simulink model "Serialising"  (R2024b)
settings: Solver=VariableStepAuto  StartTime=0.0  StopTime=10.0  RelTol=1e-3
model workspace (MAT data in the model file):
  R = 1000
libraries: hdlsllib x2
settings Model: Creator=daniel  LastModifiedBy=daniel

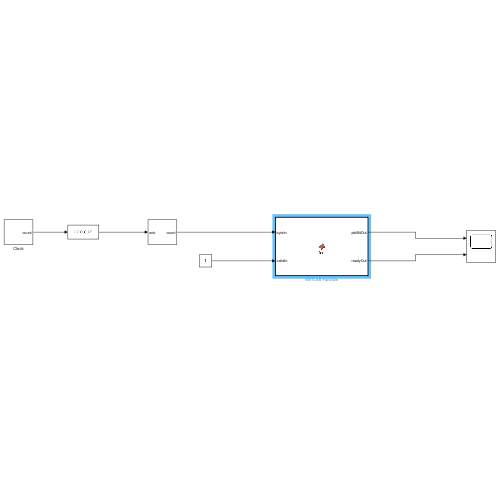
[thumbnail: Simulink's stored preview of the top-level diagram]
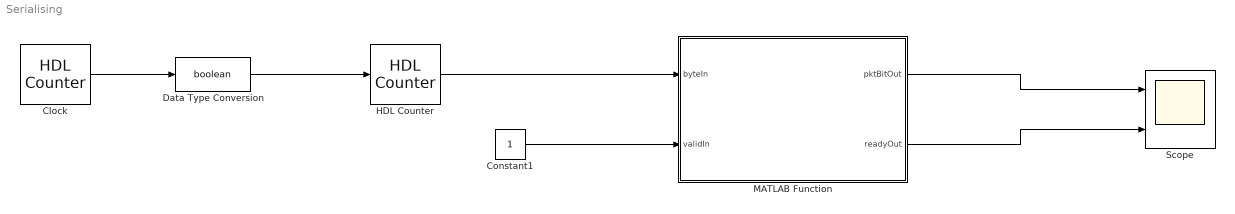
== system Serialising ==
  Clock : hdlsllib/Sources/HDL Counter  CountType=Modulo  CountInit=0  CountStep=1  CountMax=1  CountFromType=Initial value  CountFrom=0  CountResetPort=off  CountLoadPort=off  CountEnbPort=off  CountDirPort=off  CountHitOutputPort=off  CountDataType=Unsigned  CountWordLen=1  CountFracLen=0  CountSampTime=1/R
  Constant1 : Constant
  Data Type Conversion : DataTypeConversion  OutDataTypeStr=boolean  SaturateOnIntegerOverflow=off  RndMeth=Floor
  HDL Counter : hdlsllib/Sources/HDL Counter  CountType=Count limited  CountInit=0  CountStep=1  CountMax=255  CountFromType=Initial value  CountFrom=0  CountResetPort=off  CountLoadPort=off  CountEnbPort=on  CountDirPort=off  CountHitOutputPort=off  CountDataType=Unsigned  CountWordLen=8  CountFracLen=0  CountSampTime=1
  MATLAB Function : MATLAB Function  TreatAsAtomicUnit=on
  Scope : Scope  NumInputPorts=2
  wires:
  HDL Counter/1 -> MATLAB Function/1(byteIn)
  Data Type Conversion/1 -> HDL Counter/1
  Constant1/1 -> MATLAB Function/2(validIn)
  MATLAB Function/1(pktBitOut) -> Scope/1
  MATLAB Function/2(readyOut) -> Scope/2
  Clock/1 -> Data Type Conversion/1

== matlab function Serialising/MATLAB Function ==
  data: byteIn input; pktBitOut output; validIn input; readyOut output; LSBfirst parameter boolean
% Serialise 8 bit number into 8 1 bit numbers
% On Valid In & Ready: Read dataIn
% next 8 cycles: dataIn bits are output on pktBitsOut
% If no valid input: Hold current output state
function [pktBitOut,readyOut] = fcn(byteIn,validIn, LSBfirst)

    
    % Persistent Vars            
    persistent count;
    persistent byteInReg;
    if isempty(count)
        count = fi(1,0,log2(8),0,hdlfimath);
        byteInReg = fi(0,0,2,0,hdlfimath);
    end

    % Other Vars
    it = fi(1,0,log2(8),0,hdlfimath);

    % Extract bit
    switch count
        case count == 1
            if validIn
                byteInReg(:) = byteIn;
                
                if LSBfirst
                    it(:) = count;
                else
                    it(:) = 8 - (count-1);
                end
                
                readyOut = false;
                pktBitOut = bitget(byteInReg,it);
                count(:) = count + 1;
            else
                % Set Ready, wait for valid data
                count(:) = 1;
                it(:) = 1;
                readyOut = true;
                pktBitOut = bitget(byteInReg,it);

            end
        case count < 8 & count > 1
            if LSBfirst
                    it(:) = count;
                else
                    it(:) = 8 - (count-1);
                end
            pktBitOut = bitget(byteInReg,it);
            readyOut = false;
            count(:) = count + 1;            
        case count == 8
            if LSBfirst
                    it(:) = count;
                else
                    it(:) = 8 - (count-1);
                end
            pktBitOut = bitget(byteInReg,it);
            readyOut = false;
            count(:) = 1;
        otherwise
            count(:) = 1;
            it(:) = 1;
            readyOut = false;
            pktBitOut = bitget(byteInReg,it);

    end



end
